simulink model "Model"  (R2020a)
settings: Solver=VariableStepAuto  StartTime=0.0  StopTime=10.0  RelTol=1e-3
settings Model: Creator=bolt  LastModifiedBy=Khaled

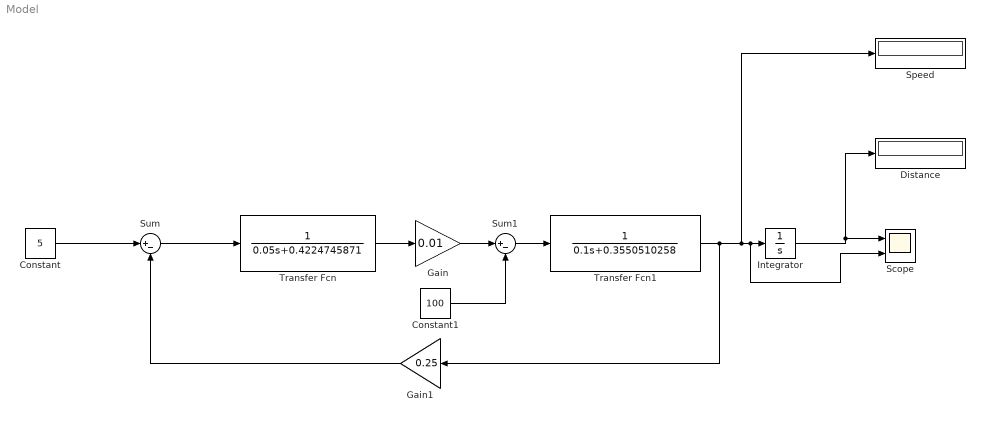
== system Model ==
  Constant : Constant  Value=5
  Constant1 : Constant  Value=100
  Distance : Display
  Gain : Gain  Gain=0.01
  Gain1 : Gain  Gain=0.25
  Integrator : Integrator
  Scope : Scope  NumInputPorts=2
  Speed : Display
  Sum : Sum  Inputs=|+-
  Sum1 : Sum  Inputs=|+-
  Transfer Fcn : TransferFcn  Denominator=[0.05 0.4224745871]
  Transfer Fcn1 : TransferFcn  Denominator=[0.1 0.3550510258]
  wires:
  Constant/1 -> Sum/1
  Sum/1 -> Transfer Fcn/1
  Transfer Fcn/1 -> Gain/1
  Gain/1 -> Sum1/1
  Constant1/1 -> Sum1/2
  Sum1/1 -> Transfer Fcn1/1
  Transfer Fcn1/1 -> Gain1/1, Speed/1, Scope/2, Integrator/1
  Gain1/1 -> Sum/2
  Integrator/1 -> Distance/1, Scope/1
